simulink model "sampleModel1613_1_sub_sub_sub"  (R2023a)
settings: Solver=VariableStepAuto  StartTime=0.0  StopTime=10.0  RelTol=1e-3
libraries: hdlsllib x5
settings Model: Creator=user1  LastModifiedBy=user1

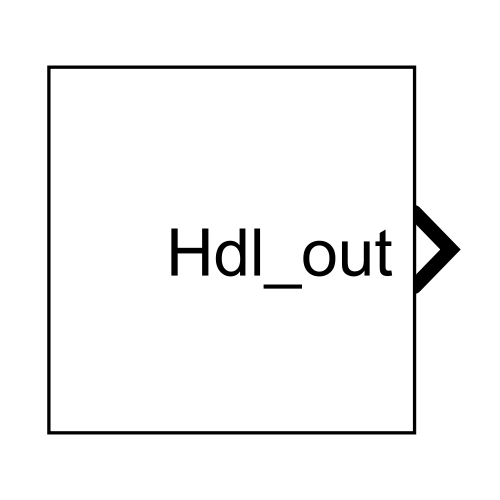
[thumbnail: Simulink's stored preview of the top-level diagram]
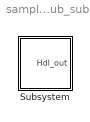
== system sampleModel1613_1_sub_sub_sub ==
  Subsystem : Subsystem

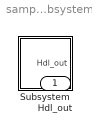
== system sampleModel1613_1_sub_sub_sub/Subsystem ==
  Subsystem : Subsystem
  Hdl_out : Outport  OutDataTypeStr=uint8

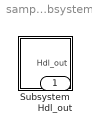
== system sampleModel1613_1_sub_sub_sub/Subsystem/Subsystem ==
  Subsystem : Subsystem
  Hdl_out : Outport  OutDataTypeStr=uint8

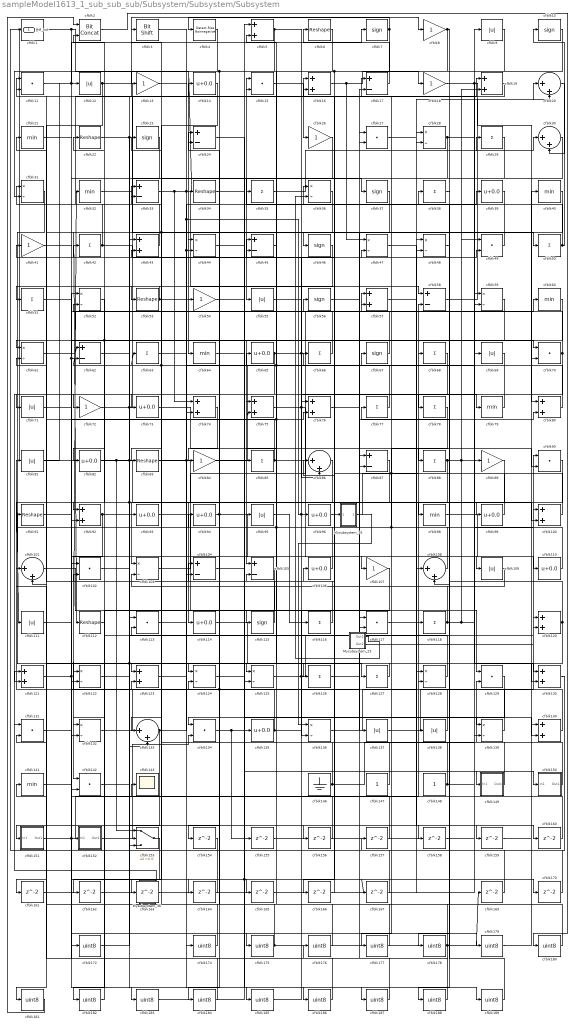
== system sampleModel1613_1_sub_sub_sub/Subsystem/Subsystem/Subsystem ==
  Mysubsystem_23 : Subsystem  TreatAsAtomicUnit=on  RTWFcnName=Mysubsystem_23
      settings: RTWFcnNameOpts=User specified  RTWFileNameOpts=Use function name
  Mysubsystem_35 : Subsystem  TreatAsAtomicUnit=on  RTWFcnName=Mysubsystem_35
      settings: RTWFcnNameOpts=User specified  RTWFileNameOpts=Use function name
  Mysubsystem_36 : Subsystem  TreatAsAtomicUnit=on  RTWFcnName=Mysubsystem_36
      settings: RTWFcnNameOpts=User specified  RTWFileNameOpts=Use function name
  cfblk1 : hdlsllib/Logic and Bit Operations/Compare To Zero  relop=<=  OutDataTypeStr=uint8
  cfblk{7,10,23,37,46,56,67,115} (8 alike) : Signum
  cfblk{5,16,19,43,57,74..76,80,92,100,120..121,123,130,140} (16 alike) : Sum  OutDataTypeStr=uint8
  cfblk{20,30,86,101,108,133} (6 alike) : Sum  Inputs=|++  OutDataTypeStr=uint8
  cfblk{11,15,27,49,70,90,102,113,117,129,131,134,142} (13 alike) : DotProduct  OutDataTypeStr=uint8
  cfblk{28,31,36,44,47..48,52,59,61,103,122,124..125,128,132,136,139} (17 alike) : Product  Inputs=*/  OutDataTypeStr=uint8  RndMeth=Zero  SaturateOnIntegerOverflow=on
  cfblk{17,24,33,45,58,62,87,104..105} (9 alike) : Sum  Inputs=+-  OutDataTypeStr=uint8
  cfblk{14,39,65,73,82,93..94,96,99,106,110,114,135} (13 alike) : Bias  Bias=0.0  SaturateOnIntegerOverflow=off
  cfblk{8,13,18,26,41,54,72,84,89,107} (10 alike) : Gain  OutDataTypeStr=uint8
  cfblk{9,12,55,69,71,81,95,109,111,137..138} (11 alike) : Abs  OutDataTypeStr=uint8  SaturateOnIntegerOverflow=off
  cfblk{6,22,34,53,83,91,112} (7 alike) : Reshape
  cfblk{29,35,38,42,50..51,63,66,68,77..78,85,88,116,118,126..127} (17 alike) : Sum  Inputs=+  OutDataTypeStr=uint8
  cfblk{21,32,40,60,64,79,98,141} (8 alike) : MinMax  OutDataTypeStr=uint8
  cfblk143 : Scope
  cfblk146 : Ground
  cfblk147 : Constant  OutDataTypeStr=uint8  SampleTime=-1
  cfblk148 : Constant  OutDataTypeStr=uint8  SampleTime=-1
  cfblk149 : Subsystem
      settings: LibrarySourceBlock=|
      | hdlsllib/Ports &
      | Subsystems/Subsystem
  cfblk150 : Subsystem
      settings: LibrarySourceBlock=|
      | hdlsllib/Ports &
      | Subsystems/Subsystem
  cfblk151 : Subsystem
      settings: LibrarySourceBlock=|
      | hdlsllib/Ports &
      | Subsystems/Subsystem
  cfblk152 : Subsystem
      settings: LibrarySourceBlock=|
      | hdlsllib/Ports &
      | Subsystems/Subsystem
  cfblk153 : Switch  OutDataTypeStr=uint8  SaturateOnIntegerOverflow=off  InputSameDT=off
  cfblk{154..167,169..170} (16 alike) : Delay  SampleTime=1
  cfblk{172,174..189} (17 alike) : DataTypeConversion  OutDataTypeStr=uint8  SaturateOnIntegerOverflow=off  RndMeth=Floor
  cfblk2 : hdlsllib/Logic and Bit Operations/Bit Concat  numInputs=2
  cfblk3 : hdlsllib/Logic and Bit Operations/Bit Shift  mode=Shift Left Logical  N=0
  cfblk4 : hdlsllib/Logic and Bit Operations/Detect Rise Nonnegative  vinit=0  OutDataTypeStr=uint8
  Hdl_out : Outport  OutDataTypeStr=uint8
  wires:
  cfblk72/1 -> cfblk164/1, cfblk19/1
  cfblk58/1 -> cfblk20/1
  cfblk17/1 -> cfblk6/1
  cfblk113/1 -> cfblk175/1
  cfblk33/1 -> cfblk74/1, cfblk58/1, cfblk70/1, Mysubsystem_35/1(In1)
  cfblk95/1 -> cfblk116/1
  cfblk59/1 -> cfblk105/1
  cfblk120/1 -> cfblk77/1, cfblk161/1, cfblk153/2
  cfblk16/1 -> cfblk47/1, cfblk18/1
  cfblk22/1 -> cfblk104/2, cfblk37/1
  cfblk94/1 -> cfblk184/1, cfblk109/1
  cfblk83/1 -> cfblk66/1, cfblk95/1
  cfblk81/1 -> cfblk12/1
  cfblk31/1 -> cfblk127/1
  cfblk53/1 -> cfblk186/1, cfblk51/1
  cfblk86/1 -> cfblk103/1
  cfblk74/1 -> cfblk84/1
  cfblk61/1 -> cfblk56/1
  cfblk29/1 -> cfblk55/1
  cfblk92/1 -> cfblk165/1, cfblk142/1
  cfblk42/1 -> cfblk47/2, cfblk8/1
  cfblk151/1(Out1) -> cfblk60/1, cfblk58/2
  cfblk46/1 -> cfblk61/1
  cfblk40/1 -> cfblk178/1
  cfblk150/1(Out1) -> cfblk106/1
  cfblk139/1 -> cfblk81/1
  cfblk88/1 -> cfblk100/2, cfblk49/1, cfblk153/3, cfblk111/1
  cfblk90/1 -> cfblk114/1
  cfblk1/1 -> cfblk179/1, cfblk64/1
  cfblk93/1 -> cfblk129/1
  cfblk98/1 -> cfblk110/1
  cfblk96/1 -> cfblk68/1
  cfblk138/1 -> cfblk24/1, cfblk32/1
  cfblk104/1 -> cfblk57/1
  cfblk125/1 -> cfblk139/1, cfblk69/1
  cfblk116/1 -> cfblk21/1
  cfblk103/1 -> cfblk27/1
  cfblk84/1 -> cfblk9/1
  cfblk50/1 -> cfblk10/1, cfblk15/1
  cfblk85/1 -> Hdl_out/1, cfblk11/1, cfblk118/1
  cfblk127/1 -> cfblk122/1
  cfblk8/1 -> cfblk13/1, cfblk78/1
  cfblk123/1 -> cfblk54/1
  cfblk106/1 -> cfblk91/1
  cfblk70/1 -> cfblk3/1, cfblk98/1
  cfblk36/1 -> cfblk83/1, cfblk112/1
  cfblk75/1 -> cfblk79/1, cfblk128/1
  cfblk136/1 -> cfblk28/2
  cfblk37/1 -> cfblk101/2
  cfblk11/1 -> cfblk70/2, cfblk7/1
  cfblk48/1 -> cfblk108/2
  cfblk26/1 -> cfblk35/1
  cfblk89/1 -> cfblk125/1
  cfblk91/1 -> cfblk142/2
  cfblk87/1 -> cfblk123/1
  cfblk5/1 -> cfblk74/2, cfblk50/1
  cfblk110/1 -> cfblk61/2
  cfblk19/1 -> cfblk15/2
  cfblk64/1 -> cfblk87/2
  cfblk118/1 -> cfblk86/1, cfblk130/1, cfblk19/2
  cfblk56/1 -> cfblk29/1
  cfblk35/1 -> cfblk30/1
  cfblk147/1 -> cfblk31/1
  cfblk27/1 -> cfblk20/2
  cfblk146/1 -> cfblk41/1, cfblk89/1
  cfblk7/1 -> cfblk4/1, cfblk44/1
  cfblk30/1 -> cfblk134/1
  cfblk121/1 -> cfblk124/2, cfblk57/2
  cfblk57/1 -> cfblk48/1
  cfblk135/1 -> cfblk24/2, cfblk49/2, cfblk96/1
  cfblk149/1(Out1) -> cfblk129/2
  cfblk133/1 -> cfblk181/1, cfblk39/1
  cfblk67/1 -> cfblk22/1
  cfblk77/1 -> cfblk45/1, cfblk62/1
  cfblk28/1 -> cfblk53/1, cfblk59/1
  cfblk114/1 -> cfblk126/1
  cfblk39/1 -> cfblk122/2
  cfblk107/1 -> cfblk132/1
  cfblk9/1 -> cfblk31/2
  cfblk21/1 -> cfblk152/1(In1)
  cfblk24/1 -> cfblk125/2
  cfblk20/1 -> cfblk30/2
  cfblk142/1 -> cfblk93/1
  cfblk54/1 -> cfblk99/1
  cfblk152/1(Out1) -> cfblk134/2
  cfblk140/1 -> cfblk16/1
  cfblk100/1 -> cfblk42/1
  cfblk124/1 -> cfblk187/1, cfblk167/1
  cfblk52/1 -> cfblk82/1
  cfblk128/1 -> cfblk52/2
  cfblk10/1 -> cfblk166/1, cfblk75/1
  cfblk49/1 -> cfblk46/1
  cfblk99/1 -> cfblk11/2, cfblk67/1
  cfblk79/1 -> cfblk73/1
  cfblk82/1 -> cfblk153/1, cfblk14/1, cfblk137/1
  cfblk111/1 -> cfblk76/2
  cfblk69/1 -> cfblk72/1
  cfblk68/1 -> cfblk115/1
  cfblk108/1 -> cfblk17/1, cfblk43/2, cfblk75/2, cfblk45/2
  cfblk12/1 -> cfblk151/1(In1), cfblk86/2
  cfblk137/1 -> cfblk120/1
  cfblk60/1 -> cfblk71/1, cfblk92/1
  cfblk148/1 -> cfblk100/1, cfblk104/1
  cfblk126/1 -> cfblk27/2
  cfblk43/1 -> cfblk33/1
  cfblk18/1 -> cfblk130/2, cfblk80/1
  cfblk132/1 -> cfblk117/1
  cfblk32/1 -> cfblk117/2
  cfblk76/1 -> cfblk80/2
  cfblk115/1 -> cfblk63/1, cfblk33/2
  cfblk45/1 -> cfblk85/1
  cfblk63/1 -> cfblk36/1, cfblk44/2
  cfblk55/1 -> cfblk90/2
  cfblk23/1 -> cfblk92/2
  cfblk109/1 -> cfblk103/2
  cfblk34/1 -> cfblk140/2
  cfblk15/1 -> cfblk26/1
  cfblk105/1 -> cfblk133/1
  cfblk122/1 -> cfblk120/2
  cfblk65/1 -> cfblk121/2, cfblk88/1, cfblk17/2
  cfblk6/1 -> cfblk124/1, cfblk34/1
  cfblk101/1 -> cfblk136/2
  cfblk4/1 -> cfblk132/2, cfblk62/2
  cfblk73/1 -> cfblk138/1
  cfblk47/1 -> cfblk150/1(In1)
  cfblk134/1 -> cfblk155/1, cfblk149/1(In1)
  cfblk66/1 -> cfblk23/1
  cfblk80/1 -> cfblk5/2
  cfblk71/1 -> cfblk107/1
  cfblk129/1 -> cfblk154/1
  cfblk154/1 -> cfblk1/1
  cfblk155/1 -> cfblk59/2
  cfblk62/1 -> cfblk156/1
  cfblk156/1 -> cfblk5/1
  cfblk130/1 -> cfblk157/1
  cfblk157/1 -> cfblk105/2
  cfblk44/1 -> cfblk158/1
  cfblk158/1 -> cfblk128/2
  cfblk117/1 -> cfblk159/1
  cfblk159/1 -> cfblk140/1
  cfblk3/1 -> cfblk160/1
  cfblk160/1 -> cfblk52/1
  cfblk161/1 -> cfblk133/2
  cfblk153/1 -> cfblk162/1
  cfblk162/1 -> cfblk108/1
  cfblk14/1 -> cfblk163/1
  cfblk163/1 -> cfblk48/2
  cfblk164/1 -> cfblk123/2
  cfblk165/1 -> cfblk139/2
  cfblk166/1 -> cfblk16/2
  cfblk167/1 -> cfblk121/1
  cfblk169/1 -> cfblk28/1
  cfblk51/1 -> cfblk170/1
  cfblk170/1 -> cfblk101/1
  cfblk131/1 -> cfblk172/1
  cfblk172/1 -> cfblk43/1
  cfblk13/1 -> cfblk174/1
  cfblk174/1 -> cfblk131/2
  cfblk175/1 -> cfblk143/1, cfblk169/1
  cfblk176/1 -> cfblk113/1
  cfblk78/1 -> cfblk177/1
  cfblk177/1 -> cfblk113/2
  cfblk178/1 -> cfblk94/1, cfblk176/1
  cfblk179/1 -> cfblk40/1
  cfblk2/1 -> cfblk180/1
  cfblk180/1 -> cfblk65/1
  cfblk181/1 -> cfblk2/1
  cfblk112/1 -> cfblk182/1
  cfblk182/1 -> cfblk2/2
  cfblk141/1 -> cfblk183/1
  cfblk183/1 -> cfblk135/1
  cfblk184/1 -> cfblk141/1
  cfblk102/1 -> cfblk185/1
  cfblk185/1 -> cfblk76/1
  cfblk186/1 -> cfblk102/1
  cfblk187/1 -> cfblk102/2
  cfblk38/1 -> cfblk188/1
  cfblk188/1 -> cfblk87/1
  cfblk41/1 -> cfblk189/1
  cfblk189/1 -> cfblk38/1
  Mysubsystem_23/1(Out1) -> cfblk36/2
  Mysubsystem_23/2(Out2) -> cfblk90/1
  Mysubsystem_35/1(Out1) -> cfblk136/1
  Mysubsystem_36/1(Out1) -> cfblk131/1

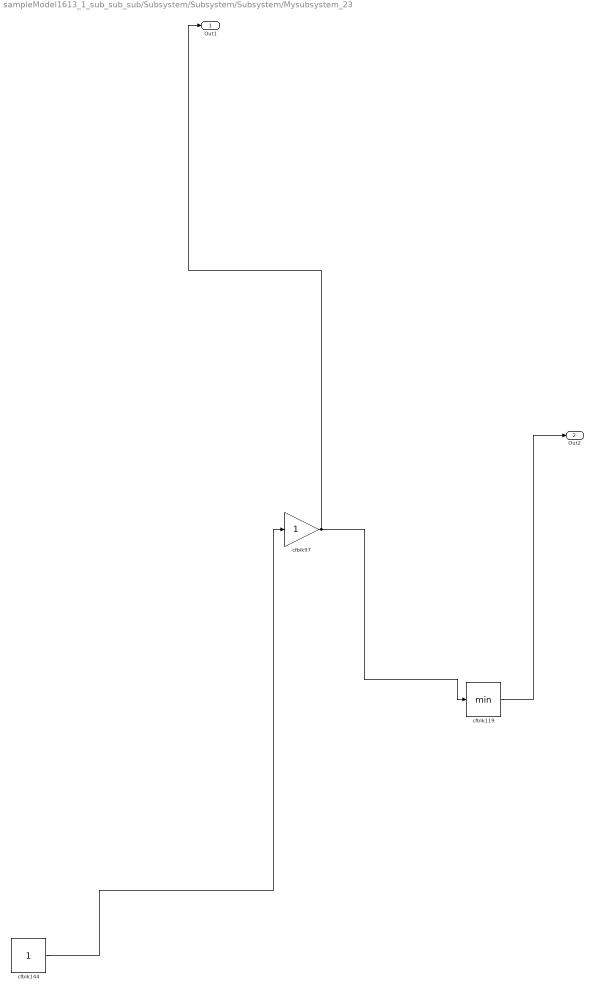
== system sampleModel1613_1_sub_sub_sub/Subsystem/Subsystem/Subsystem/Mysubsystem_23 ==
  cfblk119 : MinMax
  cfblk144 : Constant  SampleTime=-1
  cfblk97 : Gain
  Out1 : Outport
  Out2 : Outport  Port=2
  wires:
  cfblk119/1 -> Out2/1
  cfblk144/1 -> cfblk97/1
  cfblk97/1 -> cfblk119/1, Out1/1

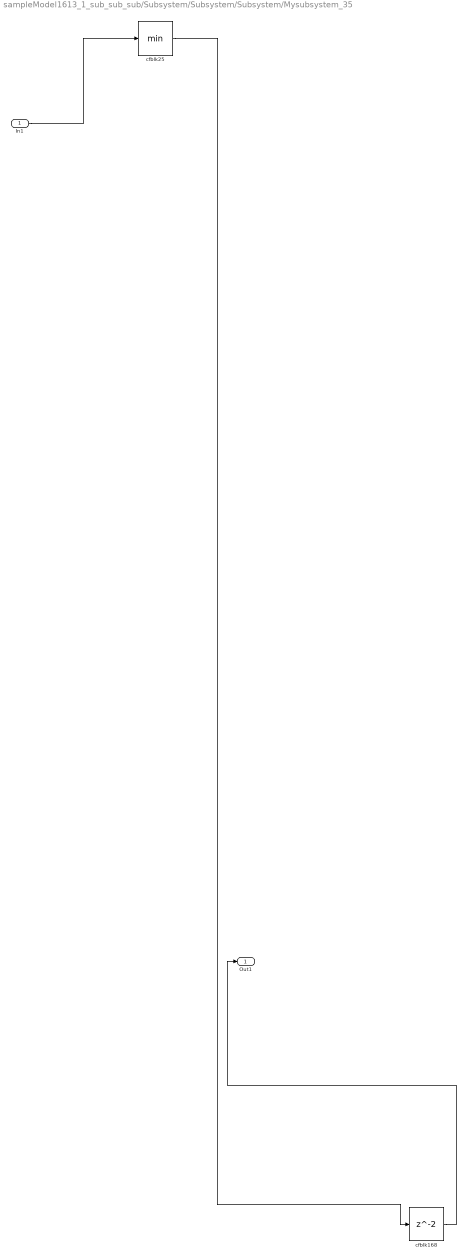
== system sampleModel1613_1_sub_sub_sub/Subsystem/Subsystem/Subsystem/Mysubsystem_35 ==
  In1 : Inport
  cfblk168 : Delay  SampleTime=1
  cfblk25 : MinMax
  Out1 : Outport
  wires:
  cfblk168/1 -> Out1/1
  In1/1 -> cfblk25/1
  cfblk25/1 -> cfblk168/1

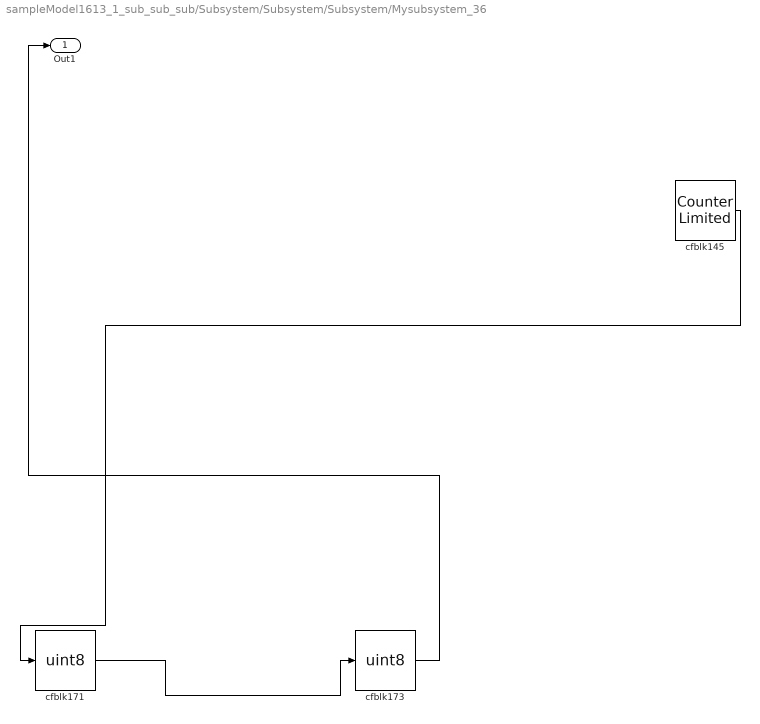
== system sampleModel1613_1_sub_sub_sub/Subsystem/Subsystem/Subsystem/Mysubsystem_36 ==
  cfblk145 : hdlsllib/Sources/Counter Limited  uplimit=7  tsamp=-1
  cfblk171 : DataTypeConversion  OutDataTypeStr=uint8  SaturateOnIntegerOverflow=off  RndMeth=Floor
  cfblk173 : DataTypeConversion  OutDataTypeStr=uint8  SaturateOnIntegerOverflow=off  RndMeth=Floor
  Out1 : Outport
  wires:
  cfblk173/1 -> Out1/1
  cfblk145/1 -> cfblk171/1
  cfblk171/1 -> cfblk173/1

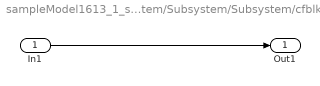
== system sampleModel1613_1_sub_sub_sub/Subsystem/Subsystem/Subsystem/cfblk149 ==
  In1 : Inport
  Out1 : Outport
  wires:
  In1/1 -> Out1/1

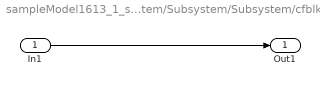
== system sampleModel1613_1_sub_sub_sub/Subsystem/Subsystem/Subsystem/cfblk150 ==
  In1 : Inport
  Out1 : Outport
  wires:
  In1/1 -> Out1/1

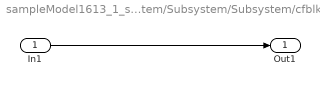
== system sampleModel1613_1_sub_sub_sub/Subsystem/Subsystem/Subsystem/cfblk151 ==
  In1 : Inport
  Out1 : Outport
  wires:
  In1/1 -> Out1/1

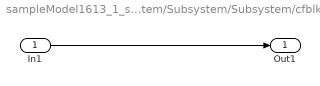
== system sampleModel1613_1_sub_sub_sub/Subsystem/Subsystem/Subsystem/cfblk152 ==
  In1 : Inport
  Out1 : Outport
  wires:
  In1/1 -> Out1/1
